simulink model "robot_assembly_Micky_torque"  (R2020a)
settings: Solver=ode4  StartTime=0.0  StopTime=Ttot  FixedStep=0.001  RelTol=1e-3
model workspace: external: MATLAB File C:\Users\miche\OneDrive - unibs.it\University\Magistrale - UNIBS\1_Primo Anno\Servosystems & Robotics\Servosystems & Robotics Project\src\Control\robot_assembly_DataFile.m (data not in the file)
undefined symbols (not defined in the file or in its folder): dT_target, Fq_interp, Q_interp, Qp_interp, Qpp_interp, smiData, X, Y, Z
libraries: sm_lib x46, nesl_utility x22
(part 2 of 2)

== matlab function robot_assembly_Micky_torque/Trajectory Generator ==
  data: t input; dT_target parameter; q1 output; q2 output; q3 output; q1p output; q2p output; q3p output; q1pp output; q2pp output; q3pp output; Q_interp parameter; Qp_interp parameter; Qpp_interp parameter; Fq1 output; Fq2 output; Fq3 output; Fq_interp parameter
function [q1,q2,q3,q1p,q2p,q3p,q1pp,q2pp,q3pp,Fq1,Fq2,Fq3] = traj_gen(t,dT_target, ...
                                    Q_interp,Qp_interp,Qpp_interp,Fq_interp)

    i = floor(t/dT_target)+1;
    i = min(i,size(Q_interp,2));
    
 
%     q1 = Q(1,i);
%     q2 = Q(2,i);
%     q3 = Q(3,i);
%     q1p = Qp(1,i);
%     q2p = Qp(2,i);
%     q3p = Qp(3,i);
%     q1pp = Qpp(1,i);
%     q2pp = Qpp(2,i);
%     q3pp = Qpp(3,i);


    q1 = Q_interp(1,i);
    q2 = Q_interp(2,i);
    q3 = Q_interp(3,i);
    q1p = Qp_interp(1,i);
    q2p = Qp_interp(2,i);
    q3p = Qp_interp(3,i);
    q1pp = Qpp_interp(1,i);
    q2pp = Qpp_interp(2,i);
    q3pp = Qpp_interp(3,i);
    
    Fq1 = Fq_interp(1,i);
    Fq2 = Fq_interp(2,i);
    Fq3 = Fq_interp(3,i);
    
end
